simulink model "simulink_commande_retour_etat"  (R2023a)
settings: Solver=VariableStepAuto  StartTime=0.0  StopTime=10.0  RelTol=1e-3
values from neighbouring files (symbols this model uses):
  K = lqr(A,B,Cksi'*Cksi,10)    [Code_main.m]
settings Model: Creator=bilheuxl  LastModifiedBy=bilheuxl

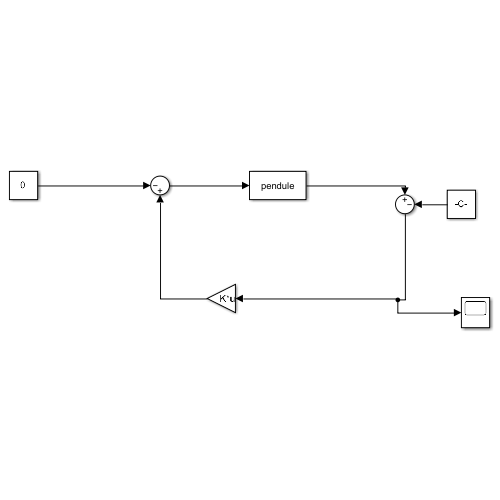
[thumbnail: Simulink's stored preview of the top-level diagram]
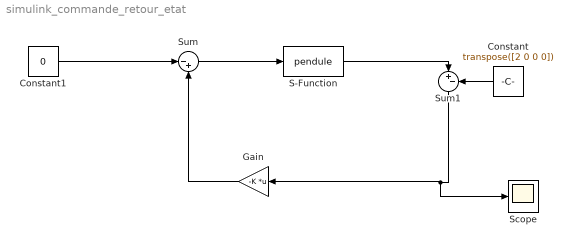
== system simulink_commande_retour_etat ==
  Constant : Constant  Value=transpose([2 0 0 0])
  Constant1 : Constant  Value=0
  Gain : Gain  Gain=-K  Multiplication=Matrix(K*u)
  S-Function : S-Function  FunctionName=pendule  SFunctionDeploymentMode=off  EnableBusSupport=off
  Scope : Scope
  Sum : Sum  Inputs=|-+
  Sum1 : Sum  Inputs=|+-
  wires:
  Sum/1 -> S-Function/1
  Constant1/1 -> Sum/1
  Gain/1 -> Sum/2
  Sum1/1 -> Scope/1, Gain/1
  Constant/1 -> Sum1/2
  S-Function/1 -> Sum1/1
